simulink model "ex_initialize_reset_terminate_henkou"  (R2019b)
settings: Solver=FixedStepDiscrete  StartTime=0.0  StopTime=20  FixedStep=1  RelTol=1e-3
undefined symbols (not defined in the file): D1, DiscIntNeverNeededParam, I, initialize, P, R, reset, T, terminate
settings Model: Creator=The MathWorks, Inc.  LastModifiedBy=I22842
settings DebuggingCC: PregeneratedLibrarySubsystemCodeDiagnostic=none  ArithmeticOperatorsInVariantConditions=warning
settings SFSimCC: SimUseLocalCustomCode=off  CustomCodeUndefinedFunction=UseInterfaceOnly
settings RTWCC: GenCodeOnly=on  GenerateReport=on  RTWUseLocalCustomCode=off  LaunchReport=on
settings CodeAppCC: StateflowObjectComments=on
settings GRTTargetCC: MatFileLogging=off  SupportNonFinite=off
settings ConfigComp: CovMetricSettings=dswe

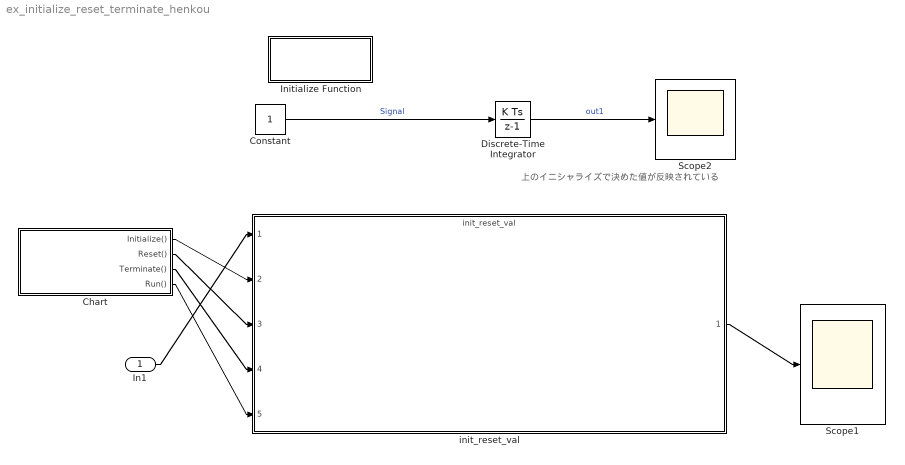
== system ex_initialize_reset_terminate_henkou ==
  note: 上のイニシャライズで決めた値が反映されている
  In1 : Inport
  Chart : Stateflow chart  BlockKeywords=__PRM__SERIALIZED__DATA__:Stateflow Chart,Stateflow Diagram  TreatAsAtomicUnit=on
  Constant : Constant
  Discrete-Time Integrator : DiscreteIntegrator  gainval=0.1  ICPrevOutput=DiscIntNeverNeededParam  ICPrevScaledInput=DiscIntNeverNeededParam
  Initialize Function : Subsystem  TreatAsAtomicUnit=on
  Scope1 : Scope
  Scope2 : Scope
  init_reset_val : ModelReference  ModelNameDialog=init_reset_val  SimulationMode=Normal  ShowModelInitializePort=on  ShowModelResetPorts=on  ShowModelTerminatePort=on  ScheduleRates=on  CachedPortDiscreteRates=[-1]  ModelEventPortInfo=I:initialize,R:reset,T:terminate,P:D1[-1][0][0]  ModelReferenceVersion=1.33
  wires:
  Chart/1(Initialize()) -> init_reset_val/2
  Chart/2(Reset()) -> init_reset_val/3
  Chart/3(Terminate()) -> init_reset_val/4
  Chart/4(Run()) -> init_reset_val/5
  init_reset_val/1 -> Scope1/1
  Constant/1 -> Discrete-Time Integrator/1  "Signal"
  Discrete-Time Integrator/1 -> Scope2/1  "out1"
  In1/1 -> init_reset_val/1

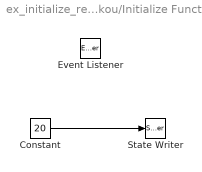
== system ex_initialize_reset_terminate_henkou/Initialize Function ==
  Constant : Constant  DisableCoverage=on  Value=20
  Event Listener : EventListener  DisableCoverage=on  EventName=reset
  State Writer : StateWriter  DisableCoverage=on  StateOwnerBlock=../../Discrete-Time Integrator
  wires:
  Constant/1 -> State Writer/1

== stateflow chart ex_initialize_reset_terminate_henkou/Chart ==
  state Inactive
    entry: step = 0;
    during: step = step + 1;
  state Running
    entry: step = step + 1; Run;
    during: step = step + 1; Run;
  (default) -> Inactive : {step = 0}
  Inactive -> Running : [step == 2]/{Initialize}
  Running -> Inactive [order 1] : [step == 9]/{Terminate}
  Running -> Running [order 2] : [step == 5]/{Reset}
  data: step local
  events: Initialize output FUNCTION_CALL_EVENT; Reset output FUNCTION_CALL_EVENT; Terminate output FUNCTION_CALL_EVENT; Run output FUNCTION_CALL_EVENT
